simulink model "Project2018"  (R2018a)
settings: Solver=ode45  StartTime=0.0  StopTime=30  MaxStep=5e-3  RelTol=1e-5  EnableMultiTasking=on
libraries: simulink x6
settings Model: Creator=tabak  LastModifiedBy=omar
settings DataIOCC: LimitDataPoints=on  SaveFormat=Array  SignalLoggingSaveFormat=ModelDataLogs
settings OptimizationCC: InitFltsAndDblsToZero=on  LifeSpan=inf
settings DebuggingCC: SaveWithParameterizedLinksMsg=none  UnderspecifiedInitializationDetection=Classic  MergeDetectMultiDrivingBlocksExec=none  SignalResolutionControl=TryResolveAllWithWarning  SolverPrmCheckMsg=warning  FcnCallInpInsideContextMsg=warning  SFUnexpectedBacktrackingDiag=warning  SFNoUnconditionalDefaultTransitionDiag=warning  SFExecutionAtInitializationDiag=none
settings HardwareCC: ProdBitPerPointer=32  ProdBitPerSizeT=32  ProdBitPerPtrDiffT=32  ProdLargestAtomicFloat=None  ProdIntDivRoundTo=Undefined  ProdEndianess=Unspecified  ProdWordSize=32  ProdHWDeviceType=32-bit Generic
settings ModelReferenceCC: PropagateSignalLabelsOutOfModel=off
settings CodeAppCC: StateflowObjectComments=on
settings GRTTargetCC: TargetFcnLib=ansi_tfl_tmw.mat  TargetLangStandard=C89/C90 (ANSI)  GeneratePreprocessorConditionals=Disable all  CombineOutputUpdateFcns=off  GRTInterface=on
settings ConfigComp: CovMetricSettings=dw  CovHtmlReporting=on  CovSaveCumulativeToWorkspaceVar=on  CovSaveSingleToWorkspaceVar=on  CovExternalEMLEnable=off  CovSFcnEnable=off

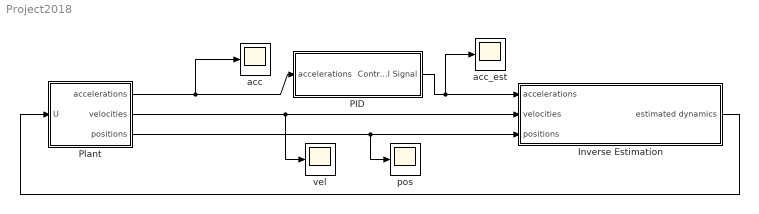
== system Project2018 ==
  Inverse Estimation : Subsystem
  PID : Subsystem
  Plant : Subsystem
  acc : Scope
  acc_est : Scope
  pos : Scope
  vel : Scope
  wires:
  Inverse Estimation/1(estimated dynamics) -> Plant/1(U)
  PID/1(Control Signal) -> Inverse Estimation/1(accelerations), acc_est/1
  Plant/1(accelerations) -> PID/1(accelerations), acc/1
  Plant/2(velocities) -> Inverse Estimation/2(velocities), vel/1
  Plant/3(positions) -> Inverse Estimation/3(positions), pos/1

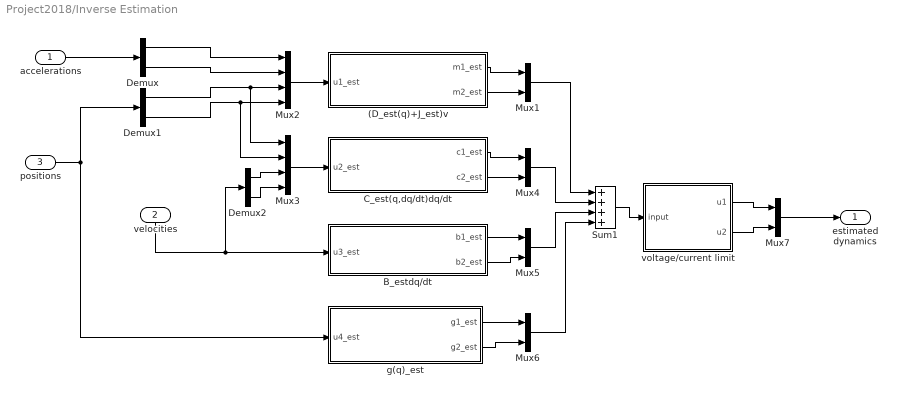
== system Project2018/Inverse Estimation ==
  accelerations : Inport
  velocities : Inport  Port=2
  positions : Inport  Port=3
  (D_est(q)+J_est)v : MATLAB Function  TreatAsAtomicUnit=on
  B_estdq/dt : MATLAB Function  TreatAsAtomicUnit=on
  C_est(q,dq/dt)dq/dt : MATLAB Function  TreatAsAtomicUnit=on
  Demux : Demux  Outputs=2
  Demux1 : Demux  Outputs=2
  Demux2 : Demux  Outputs=2
  Mux{1,4..7} (5 alike) : Mux  Inputs=2
  Mux2 : Mux
  Mux3 : Mux
  Sum1 : Sum  Inputs=++++
  g(q)_est : MATLAB Function  TreatAsAtomicUnit=on
  voltage/current limit : MATLAB Function  TreatAsAtomicUnit=on
  estimated dynamics : Outport
  wires:
  Mux2/1 -> (D_est(q)+J_est)v/1(u1_est)
  Mux3/1 -> C_est(q,dq/dt)dq/dt/1(u2_est)
  Sum1/1 -> voltage/current limit/1(input)
  g(q)_est/1(g1_est) -> Mux6/1
  B_estdq/dt/1(b1_est) -> Mux5/1
  B_estdq/dt/2(b2_est) -> Mux5/2
  C_est(q,dq/dt)dq/dt/2(c2_est) -> Mux4/2
  C_est(q,dq/dt)dq/dt/1(c1_est) -> Mux4/1
  (D_est(q)+J_est)v/2(m2_est) -> Mux1/2
  (D_est(q)+J_est)v/1(m1_est) -> Mux1/1
  Mux1/1 -> Sum1/1
  Mux4/1 -> Sum1/2
  Mux5/1 -> Sum1/3
  Mux6/1 -> Sum1/4
  g(q)_est/2(g2_est) -> Mux6/2
  positions/1 -> g(q)_est/1(u4_est), Demux1/1
  Mux7/1 -> estimated dynamics/1
  voltage/current limit/1(u1) -> Mux7/1
  voltage/current limit/2(u2) -> Mux7/2
  velocities/1 -> B_estdq/dt/1(u3_est), Demux2/1
  accelerations/1 -> Demux/1
  Demux/1 -> Mux2/1
  Demux/2 -> Mux2/2
  Demux1/1 -> Mux2/3, Mux3/1
  Demux1/2 -> Mux2/4, Mux3/2
  Demux2/1 -> Mux3/3
  Demux2/2 -> Mux3/4

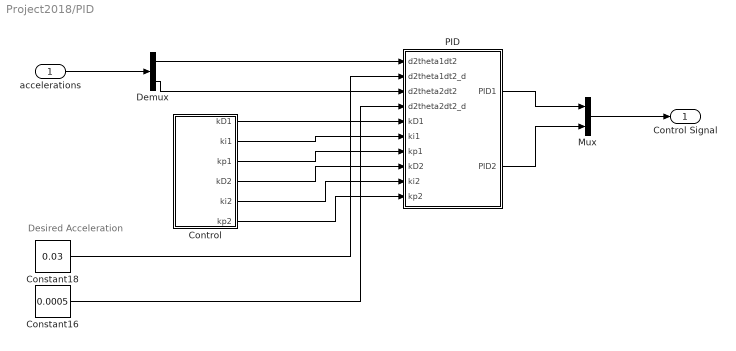
== system Project2018/PID ==
  note: Desired Acceleration
  accelerations : Inport
  Constant16 : Constant  Value=0.0005
  Constant18 : Constant  Value=0.03
  Control : Subsystem
  Demux : Demux  Outputs=2
  Mux : Mux  Inputs=2
  PID : Subsystem
  Control Signal : Outport
  wires:
  accelerations/1 -> Demux/1
  Demux/1 -> PID/1(d2theta1dt2)
  Demux/2 -> PID/3(d2theta2dt2)
  Control/1(kD1) -> PID/5(kD1)
  Control/2(ki1) -> PID/6(ki1)
  Control/3(kp1) -> PID/7(kp1)
  Control/4(kD2) -> PID/8(kD2)
  Control/5(ki2) -> PID/9(ki2)
  Control/6(kp2) -> PID/10(kp2)
  Constant18/1 -> PID/2(d2theta1dt2_d)
  Constant16/1 -> PID/4(d2theta2dt2_d)
  PID/1(PID1) -> Mux/1
  PID/2(PID2) -> Mux/2
  Mux/1 -> Control Signal/1

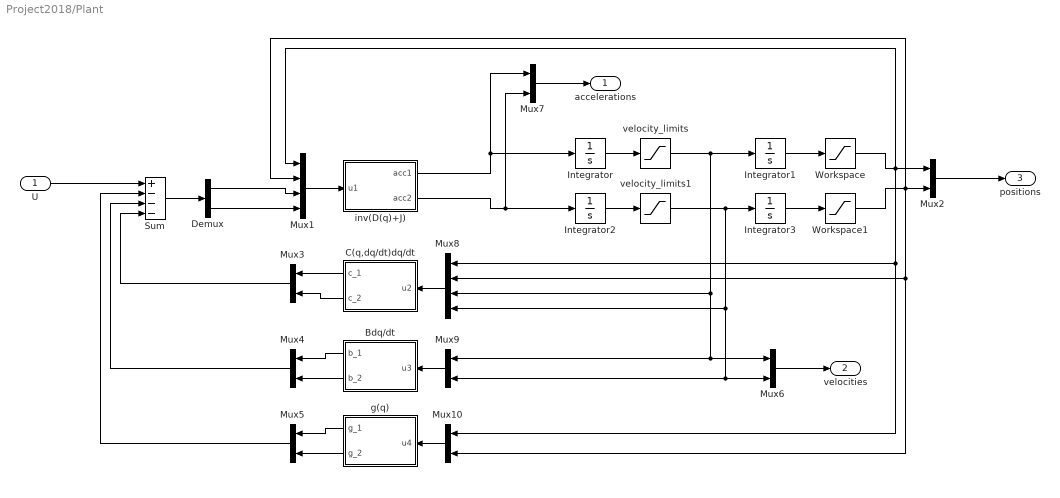
== system Project2018/Plant ==
  U : Inport
  Bdq/dt : MATLAB Function  TreatAsAtomicUnit=on
  C(q,dq/dt)dq/dt : MATLAB Function  TreatAsAtomicUnit=on
  Demux : Demux  Outputs=2
  Integrator{,1..3} (4 alike) : Integrator
  Mux1 : Mux
  Mux{2..7,9..10} (8 alike) : Mux  Inputs=2
  Mux8 : Mux
  Sum : Sum  Inputs=+---
  Workspace : Saturate  UpperLimit=1.2*(2*pi)/3  LowerLimit=-1.2*(2*pi)/3
  Workspace1 : Saturate  UpperLimit=1.2*(2*pi)/3  LowerLimit=-1.2*(2*pi)/3
  g(q) : MATLAB Function  TreatAsAtomicUnit=on
  inv(D(q)+J) : MATLAB Function  TreatAsAtomicUnit=on
  velocity_limits : Saturate  UpperLimit=1640*2*pi/60  LowerLimit=-1640*2*pi/60
  velocity_limits1 : Saturate  UpperLimit=1640*2*pi/60  LowerLimit=-1640*2*pi/60
  accelerations : Outport
  velocities : Outport  Port=2
  positions : Outport  Port=3
  wires:
  Integrator/1 -> velocity_limits/1
  Integrator1/1 -> Workspace/1
  Mux1/1 -> inv(D(q)+J)/1(u1)
  U/1 -> Sum/1
  C(q,dq/dt)dq/dt/2(c_2) -> Mux3/2
  C(q,dq/dt)dq/dt/1(c_1) -> Mux3/1
  Bdq/dt/1(b_1) -> Mux4/1
  Bdq/dt/2(b_2) -> Mux4/2
  g(q)/1(g_1) -> Mux5/1
  g(q)/2(g_2) -> Mux5/2
  Mux3/1 -> Sum/4
  Mux4/1 -> Sum/3
  Mux5/1 -> Sum/2
  velocity_limits/1 -> Integrator1/1, Mux8/3, Mux9/1, Mux6/1
  Integrator2/1 -> velocity_limits1/1
  Integrator3/1 -> Workspace1/1
  velocity_limits1/1 -> Integrator3/1, Mux8/4, Mux9/2, Mux6/2
  inv(D(q)+J)/1(acc1) -> Integrator/1, Mux7/1
  inv(D(q)+J)/2(acc2) -> Integrator2/1, Mux7/2
  Workspace/1 -> Mux2/1, Mux1/1, Mux8/1, Mux10/1
  Workspace1/1 -> Mux2/2, Mux1/2, Mux8/2, Mux10/2
  Mux2/1 -> positions/1
  Mux6/1 -> velocities/1
  Mux7/1 -> accelerations/1
  Mux8/1 -> C(q,dq/dt)dq/dt/1(u2)
  Sum/1 -> Demux/1
  Demux/2 -> Mux1/4
  Demux/1 -> Mux1/3
  Mux9/1 -> Bdq/dt/1(u3)
  Mux10/1 -> g(q)/1(u4)

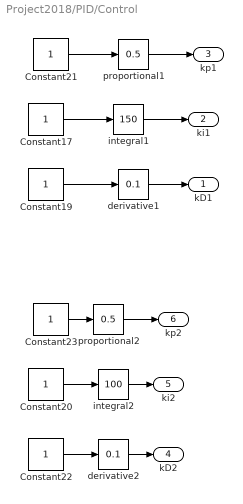
== system Project2018/PID/Control ==
  Constant{17,19..23} (6 alike) : Constant
  derivative1 : simulink/Math Operations/Slider Gain  gain=0.1  low=0  high=150
  derivative2 : simulink/Math Operations/Slider Gain  gain=0.1  low=0  high=150
  integral1 : simulink/Math Operations/Slider Gain  gain=150  low=0  high=500
  integral2 : simulink/Math Operations/Slider Gain  gain=100  low=0  high=500
  proportional1 : simulink/Math Operations/Slider Gain  gain=0.5  low=0  high=1500
  proportional2 : simulink/Math Operations/Slider Gain  gain=0.5  low=0  high=1000
  kD1 : Outport
  ki1 : Outport  Port=2
  kp1 : Outport  Port=3
  kD2 : Outport  Port=4
  ki2 : Outport  Port=5
  kp2 : Outport  Port=6
  wires:
  Constant19/1 -> derivative1/1
  Constant17/1 -> integral1/1
  Constant21/1 -> proportional1/1
  Constant22/1 -> derivative2/1
  Constant20/1 -> integral2/1
  Constant23/1 -> proportional2/1
  proportional1/1 -> kp1/1
  integral1/1 -> ki1/1
  derivative1/1 -> kD1/1
  proportional2/1 -> kp2/1
  integral2/1 -> ki2/1
  derivative2/1 -> kD2/1

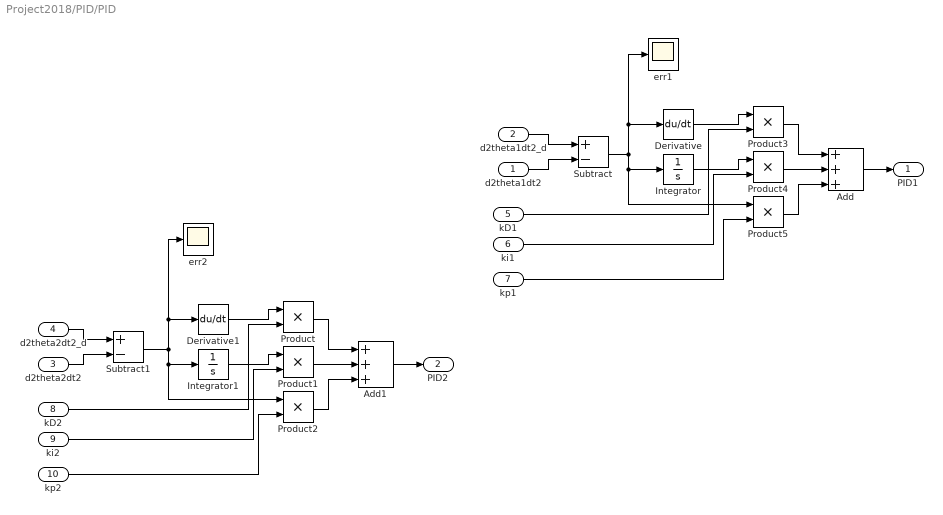
== system Project2018/PID/PID ==
  d2theta1dt2 : Inport
  d2theta1dt2_d : Inport  Port=2
  d2theta2dt2 : Inport  Port=3
  d2theta2dt2_d : Inport  Port=4
  kD1 : Inport  Port=5
  ki1 : Inport  Port=6
  kp1 : Inport  Port=7
  kD2 : Inport  Port=8
  ki2 : Inport  Port=9
  kp2 : Inport  Port=10
  Add : Sum  Inputs=+++
  Add1 : Sum  Inputs=+++
  Derivative : Derivative
  Derivative1 : Derivative
  Integrator : Integrator
  Integrator1 : Integrator
  Product{,1..5} (6 alike) : Product  RndMeth=Zero
  Subtract : Sum  Inputs=+-
  Subtract1 : Sum  Inputs=+-
  err1 : Scope
  err2 : Scope
  PID1 : Outport
  PID2 : Outport  Port=2
  wires:
  d2theta1dt2_d/1 -> Subtract/1
  d2theta1dt2/1 -> Subtract/2
  d2theta2dt2_d/1 -> Subtract1/1
  d2theta2dt2/1 -> Subtract1/2
  Subtract/1 -> Integrator/1, Product5/1, err1/1, Derivative/1
  Integrator/1 -> Product4/1
  Subtract1/1 -> Integrator1/1, Product2/1, err2/1, Derivative1/1
  Integrator1/1 -> Product1/1
  Add1/1 -> PID2/1
  Add/1 -> PID1/1
  Product4/1 -> Add/2
  Product5/1 -> Add/3
  Product1/1 -> Add1/2
  Product2/1 -> Add1/3
  kD1/1 -> Product3/2
  ki1/1 -> Product4/2
  kp1/1 -> Product5/2
  kD2/1 -> Product/2
  ki2/1 -> Product1/2
  kp2/1 -> Product2/2
  Product3/1 -> Add/1
  Product/1 -> Add1/1
  Derivative1/1 -> Product/1
  Derivative/1 -> Product3/1

== matlab function Project2018/Plant/C(q,dq/dt)dq/dt ==
  data: u2 input; c_1 output; c_2 output
function [c_1, c_2] = fcn2(u2)
% This block supports an embeddable subset of the MATLAB language.
% See the help menu for details. 

if length(u2) == 4

pos2 = u2(2); % second actuator position
vel1 = u2(3); % first actuator velocity
vel2 = u2(4); % second actuator velocity

% Link 1 
I133 = 0.000891271;
L1 = 0.2;
Lc1 = 0.1;
m1 = 0.358306058;
% Link 2 
I233 = 0.000552127;
L2 = 0.2;
Lc2 = 0.073;
m2 = 0.308756558;

% matrix variables
c111 = 0;
c112 = m2*L1*Lc2*sin(pos2);
c121 = -c112;
c211 = -c112;
c122 = 0;
c212 = 0;
c221 = -c112;
c222 = 0;

C = [(c111*vel1 +c211*vel2) (c121*vel1 +c221*vel2);...
    (c112*vel1 +c212*vel2) (c122*vel1 +c222*vel2)]; % C (2x2) matrix

Cmul = C*[vel1; vel2];

c_1 = Cmul(1,:);
c_2 = Cmul(2,:);

else
    
c_1 = 0;
c_2 = 0;
    
end

== matlab function Project2018/Plant/inv(D(q)+J) ==
  data: u1 input; acc1 output; acc2 output
function [acc1, acc2] = fcn1(u1)
% This block supports an embeddable subset of the MATLAB language.
% See the help menu for details. 

% the input U(t) is the net torque on the joints after motor and link
% variables are all accounted for.

if length(u1) == 4
    
    pos2 = u1(2); % second actuator position
    cbg1 = u1(3); % array element to be multiplied with inv(M)
    cbg2 = u1(4); % array element to be multiplied with inv(M)

    % motor variables
    j1 = 3060e-7; % rotor inertia
    j2 = j1; % rotor inertia

    % Link 1 
    I133 = 0.000891271;
    L1 = 0.2;
    Lc1 = 0.1;
    m1 = 0.358306058;
    % Link 2 
    I233 = 0.000552127;
    L2 = 0.2;
    Lc2 = 0.073;
    m2 = 0.308756558;

    % external variables
    r1 = 1/4; % first actuator reduction
    r2 = 1/3; % second actuator reduction

    % matrix variables
    d11 = m1*Lc1^2 + m2*(L1^2 +Lc2^2 +2*L1*Lc2*cos(pos2)) + I133 +I233;
    d12 = m2*(Lc2^2 +L1*Lc2*cos(pos2)) +I233;
    d21 = m2*(Lc2^2 +L1*Lc2*cos(pos2)) +I233;
    d22 = m2*Lc2^2 +I233;
    j11 = 1/(r1^2)*j1;
    j22 = 1/(r2^2)*j2;

    M = [(d11 +j11) d12; d21 (d22 +j22)]; % D(q)+J/r^2  (2x2) matrix

    accel = inv(M)*[cbg1; cbg2]; %#ok<MINV>

    acc1 = accel(1,:);
    acc2 = accel(2,:);

else
    
    acc1 = 0;
acc2 = 0;

end

== matlab function Project2018/Plant/Bdq/dt ==
  data: u3 input; b_1 output; b_2 output
function [b_1, b_2] = fcn3(u3)
% This block supports an embeddable subset of the MATLAB language.
% See the help menu for details.

if length(u3) == 2
    
    vel1 = u3(1); % first actuator velocity
    vel2 = u3(2); % second actuator velocity
    
    % motor variables
    kb = 1/(44*2*pi/60); % back emf constant
    km = 217e-3; % torque constant
    r = 2.30; % motor resistance
    mt = 14.9e-3; % mechanical time constant
    j1 = 3060e-7; % rotor inertia
    b1 = mt*j1; % motor friction
    b2 = b1; % motor friction
    
    % external variables
    r1 = 1/4; % first actuator reduction
    r2 = 1/3; % second actuator reduction
    
    % matrix variables
    b1 = 1/(r1^2)*(b1 +km*kb/r);
    b2 = 1/(r2^2)*(b2 +km*kb/r);
    
    B = [b1 0; 0 b2];
    
    Bmul = B*[vel1; vel2];
    
    b_1 = Bmul(1,:);
    b_2 = Bmul(2,:);
    
else
    
    b_1 = 0;
    b_2 = 0;
    
end

== matlab function Project2018/Plant/g(q) ==
  data: u4 input; g_1 output; g_2 output
function [g_1, g_2] = fcn4(u4)
% This block supports an embeddable subset of the MATLAB language.
% See the help menu for details.

if length(u4) == 2
    
    pos1 = u4(1); % first actuator position
    pos2 = u4(2); % second actuator position
    
    % link variables
    % Link 1 
    I133 = 0.000891271;
    L1 = 0.2;
    Lc1 = 0.1;
    m1 = 0.358306058;
    % Link 2 
    I233 = 0.000552127;
    L2 = 0.2;
    Lc2 = 0.073;
    m2 = 0.308756558;
    
    % external variables
    g = 9.81; % gravitational acceleration
    
    % matrix variables
    phi1 = (m1*Lc1 +m2*L1)*g*cos(pos1) +m2*g*Lc2*cos(pos1 +pos2);
    phi2 = m2*Lc2*cos(pos1 +pos2);
    
    g_1 = phi1;
    g_2 = phi2;
    
else
    
    g_1 = 0;
    g_2 = 0;
    
end

== matlab function Project2018/Inverse Estimation/(D_est(q)+J_est)v ==
  data: u1_est input; m1_est output; m2_est output
function [m1_est, m2_est] = fcn1_est(u1_est)
% This block supports an embeddable subset of the MATLAB language.
% See the help menu for details.

if length(u1_est) == 4
    
    % error margin
    err = 1.01; % error for everything
    
    acc1_est = u1_est(1); % estimated acceleration for first actuator
    acc2_est = u1_est(2); % estimated acceleration for second actuator
    pos2 = err*u1_est(4); % second actuator position with noise
    
    % motor variables
    j1 = err*3060e-7; % rotor inertia
    j2 = j1; % rotor inertia
    
    % Link 1 
    I133 = err*0.000891271;
    L1 = err*0.2;
    Lc1 = err*0.1;
    m1 = err*0.358306058;
    % Link 2 
    I233 = err*0.000552127;
    L2 = err*0.2;
    Lc2 = err*0.073;
    m2 = err*0.308756558;
    
    % external variables
    r1 = err*1/4; % first actuator reduction
    r2 = err*1/3; % second actuator reduction
    
    % matrix variables
    d11_est = m1*Lc1^2 + m2*(L1^2 +Lc2^2 +2*L1*Lc2*cos(pos2)) + I133 +I233;
    d12_est = m2*(Lc2^2 +L1*Lc2*cos(pos2)) +I233;
    d21_est = m2*(Lc2^2 +L1*Lc2*cos(pos2)) +I233;
    d22_est = m2*Lc2^2 +I233;
    j11_est = 1/(r1^2)*j1;
    j22_est = 1/(r2^2)*j2;
    
    M_est = [(d11_est +j11_est) d12_est;...
        d21_est (d22_est +j22_est)]; % D(q)+J/r^2  (2x2) matrix
    
    Mmul = M_est*[acc1_est; acc2_est];
    
    m1_est = Mmul(1,:);
    m2_est = Mmul(2,:);
    
else
    
    m1_est = 0;
    m2_est = 0;
    
end

== matlab function Project2018/Inverse Estimation/C_est(q,dq/dt)dq/dt ==
  data: u2_est input; c1_est output; c2_est output
function [c1_est, c2_est] = fcn2_est(u2_est)
% This block supports an embeddable subset of the MATLAB language.
% See the help menu for details.

if length(u2_est) == 4
    
    % error margin
    err = 1.01; % error for everything
    
    pos2 = err*u2_est(2); % second actuator position
    vel1 = err*u2_est(3); % first actuator velocity
    vel2 = err*u2_est(4); % second actuator velocity
    
    % Link 1 
    I133 = err*0.000891271;
    L1 = err*0.2;
    Lc1 = err*0.1;
    m1 = err*0.358306058;
    % Link 2 
    I233 = err*0.000552127;
    L2 = err*0.2;
    Lc2 = err*0.073;
    m2 = err*0.308756558;
    
    % matrix variables
    c111_est = 0;
    c112_est = m2*L1*Lc2*sin(pos2);
    c121_est = -c112_est;
    c211_est = -c112_est;
    c122_est = 0;
    c212_est = 0;
    c221_est = -c112_est;
    c222_est = 0;
    
    C_est = [(c111_est*vel1 +c211_est*vel2) (c121_est*vel1 +c221_est*vel2); ...
        (c112_est*vel1 +c212_est*vel2) (c122_est*vel1 +c222_est*vel2)]; % C (2x2) matrix
    
    Cmul_est = C_est*[vel1; vel2];
    
    c1_est = Cmul_est(1,:);
    c2_est = Cmul_est(2,:);
    
else
    
    c1_est = 0;
    c2_est = 0;
    
end

== matlab function Project2018/Inverse Estimation/B_estdq/dt ==
  data: u3_est input; b1_est output; b2_est output
function [b1_est, b2_est] = fcn3_est(u3_est)
% This block supports an embeddable subset of the MATLAB language.
% See the help menu for details.

if length(u3_est) == 2
    
    % error margin
    err = 1.01; % error for everything
    
    vel1 = err*u3_est(1); % first actuator velocity
    vel2 = err*u3_est(2); % second actuator velocity
    
    % motor variables
    kb = err*1/(44*2*pi/60); % back emf constant
    km = err*217e-3; % torque constant
    r = err*2.30; % motor resistance
    mt = err*14.9e-3; % mechanical time constant
    j1 = err*3060e-7; % rotor inertia
    b1 = mt*j1; % motor friction
    b2 = b1; % motor friction
    
    % external variables
    r1 = err*1/4; % first actuator reduction
    r2 = err*1/3; % second actuator reduction
    
    % matrix variables
    b1_est = 1/(r1^2)*(b1 +km*kb/r);
    b2_est = 1/(r2^2)*(b2 +km*kb/r);
    
    B_est = [b1_est 0; 0 b2_est];
    
    Bmul_est = B_est*[vel1; vel2];
    
    b1_est = Bmul_est(1,:);
    b2_est = Bmul_est(2,:);
    
else
    
    b1_est = 0;
    b2_est = 0;
    
end

== matlab function Project2018/Inverse Estimation/g(q)_est ==
  data: u4_est input; g1_est output; g2_est output
function [g1_est, g2_est] = fcn4_est(u4_est)
% This block supports an embeddable subset of the MATLAB language.
% See the help menu for details.

if length(u4_est) == 2
    
    % error margin
    err = 1.01; % error for everything
    
    pos1 = err*u4_est(1); % first actuator position
    pos2 = err*u4_est(2); % second actuator position
    
    % Link 1 
    I133 = err*0.000891271;
    L1 = err*0.2;
    Lc1 = err*0.1;
    m1 = err*0.358306058;
    % Link 2 
    I233 = err*0.000552127;
    L2 = err*0.2;
    Lc2 = err*0.073;
    m2 = err*0.308756558;
    
    % external variables
    g = err*9.81; % gravitational acceleration
    
    % matrix variables
    phi1_est = (m1*Lc1 +m2*L1)*g*cos(pos1) +m2*g*Lc2*cos(pos1 +pos2);
    phi2_est = m2*Lc2*cos(pos1 +pos2);
    
    g1_est = phi1_est;
    g2_est = phi2_est;
    
else
    
    g1_est = 0;
    g2_est = 0;
    
end

== matlab function Project2018/Inverse Estimation/voltage/current limit ==
  data: input input; u1 output; u2 output
function [u1, u2] = limit(input)
% This block supports an embeddable subset of the MATLAB language.
% See the help menu for details. 

% Here we estimate the required voltage! In this example, the controller 
% works on accelerations, not directly on the voltage. The reason is, the
% controller can suddenly estimate excessive/impossible/dangerous voltages. 

if length(input) == 2

u1 = input(1);
u2 = input(2);

% error margin
err = 1.01; % error for everything

% motor variables
km = err*217e-3; % torque constant
r = err*2.30; % motor resistance

% external variables
r1 = err*1/4; % first actuator reduction
r2 = err*1/3; % second actuator reduction

% volt limits
vlim = 48; % absolute limit

volt1 = u1*r1*r/km;
volt2 = u2*r2*r/km;

if volt1 >= vlim
    volt1 = vlim;
elseif volt1 <= -vlim
    volt1 = -vlim;
else
    volt1 = volt1; %#ok<ASGSL>
end

if volt2 >= vlim
    volt2 = vlim;
elseif volt2 <= -vlim
    volt2 = -vlim;
else
    volt2 = volt2; %#ok<ASGSL>
end

u1 = volt1*km/(r*r1);
u2 = volt2*km/(r*r2);

else
    
    u1 = 0;
u2 = 0;

end
